simulink model "Lidar_System_FullStateOct25"  (Simulink 7.3)
settings: Solver=FixedStepDiscrete  StartTime=0.0  StopTime=inf  FixedStep=0.1  MaxStep=0.2  RelTol=1e-3
undefined symbols (not defined in the file): strel
libraries: dspmtrx3 x28, simulink x13, dspstat3 x10, vipstatistics x7, vipmorphops x7, dspindex x1
(part 3 of 3)

== matlab function Enabled Subsystem1/Perception/Color Analysis/Docking (Circle)/Docking1/Recognition/Embedded MATLAB Function ==
  data: targetTemp input double; bbox_out output double; cruciform input double; circle input double; triangle input double; whitePixCount input double; threshold input double; V_mask input double; bbox_in input double; returnRatioDiff output double
function [bbox_out,returnRatioDiff] = recognition(targetTemp,cruciform,circle,triangle,...
    whitePixCount,threshold,V_mask,bbox_in)

% Written by Edward Zhu on 5/14/14

% Inputs
% tempID:       Number corresponding to one of the templates (cruciform: 1,
%               circle: 2, triangle: 3)
% cruciform:    19*19 template of cruciform
% circle:       19*19 template of circle
% triangle:     19*19 template of triangle
% whitePixCount:Number of white pixels in each of the templates
% V_mask:       V channel binary mask
% bbox_in:      Bounding boxes as found by blob analysis
% label:        Label matrix as found by blob analysis

% Outputs
% bbox_out:     Bounding box of matched symbol
% symFound:     Status of matching (found: 1, not found: 0)

% Define frame and template size
templates = zeros(19,19,3);
templates(:,:,1) = cruciform;
templates(:,:,2) = circle;
templates(:,:,3) = triangle;
templates = 2*(templates-0.5);

tempRows = size(templates,1);
tempCols = size(templates,2);
numBBox = size(bbox_in,1);

% Initialize scaled image and output bbox matrices
V_scaled = zeros(tempRows,tempCols);
bbox_out = uint32(zeros(numBBox,4));

returnRatioDiff = ones(numBBox,1);

for i = 1:numBBox
       
    if (min(bbox_in(i,:)) > 0 && (bbox_in(i,1)+bbox_in(i,3)) < 640  && (bbox_in(i,2) + bbox_in(i,4) < 480))
        similarity = 0;
        rowScaleStep = floor(bbox_in(i,4) / tempRows);
        colScaleStep = floor(bbox_in(i,3) / tempCols);
        
        captureRow = bbox_in(i,2);
        for row = 1:tempRows
            captureCol = bbox_in(i,1);
            if (captureCol > 640)
                captureCol = uint32(640);
            end
            if (captureRow > 480)
                captureRow = uint32(480);
            end
            for col = 1:tempCols
                V_scaled(row,col) = V_mask(captureRow,captureCol);
                similarity = similarity + templates(row,col,targetTemp) * (V_mask(captureRow,captureCol)*(-1) + 1);
                captureCol = captureCol + colScaleStep;
            end
            captureRow = captureRow + rowScaleStep;
        end
        
        ratioDiff = abs(1 - single(similarity) / single(whitePixCount(targetTemp)));
        
        % Output valid bounding box
        if ratioDiff < threshold
            bbox_out(i,:) = bbox_in(i,:);
            returnRatioDiff(i) = ratioDiff;
        end
    end
end

== matlab function Enabled Subsystem1/Perception/Color Analysis/Docking (Cross)/Docking1/Embedded MATLAB Function ==
  data: xRec input double; bayNumber output double; xDet input double
function bayNumber = bayPosition(xRec,xDet)

symxpos = xRec(1);

diff1 = xDet(1) - symxpos;
diff2 = xDet(2) - symxpos;
diff3 = xDet(3) - symxpos;

if diff1 == 0
    bayNumber = uint8(1);
elseif diff2 == 0
    bayNumber = uint8(2);
elseif diff3 == 0
    bayNumber = uint8(3);
else
    bayNumber = uint8(0);
end

== matlab function Enabled Subsystem1/Perception/Color Analysis/Docking (Cross)/Docking1/Embedded MATLAB Function1 ==
  data: uv_d input double; Distances output double; BBox input double; Angles output double
function [Distances, Angles]  = DsitFind(uv_d,BBox)

% Based on the location of the signs find their distance

% Predefine output distance matrix
Distances = zeros(4,1);
Angles = zeros(4,1);

% Parse BBox information
xpos = BBox(1,1);
ypos = BBox(1,2);
width = BBox(1,3);
height = BBox(1,4);

% Zero count and total of distance measurements
count = 0;
total = 0;

for i = ypos:(ypos+height)
    for j = xpos:(xpos+width)
        % Find total number of points in box where distance value has
        % been gathered and total of all distance in box
        if (uv_d(i,j) > 1)
            count = count+1;
            total = total+uv_d(i,j);
        end
    end
end

% Find average value of nonzero elements inside BBox
Distances(1,1) = round(total/(count*10));
Angles(1,1) = ((xpos + width)/2-3.135858904821101e+02)/554.8582*180/pi;


end

== matlab function Enabled Subsystem1/Perception/Color Analysis/Docking (Cross)/Docking1/Recognition/Embedded MATLAB Function ==
  data: targetTemp input double; bbox_out output double; cruciform input double; circle input double; triangle input double; whitePixCount input double; threshold input double; V_mask input double; bbox_in input double; returnRatioDiff output double
function [bbox_out,returnRatioDiff] = recognition(targetTemp,cruciform,circle,triangle,...
    whitePixCount,threshold,V_mask,bbox_in)

% Written by Edward Zhu on 5/14/14

% Inputs
% tempID:       Number corresponding to one of the templates (cruciform: 1,
%               circle: 2, triangle: 3)
% cruciform:    19*19 template of cruciform
% circle:       19*19 template of circle
% triangle:     19*19 template of triangle
% whitePixCount:Number of white pixels in each of the templates
% V_mask:       V channel binary mask
% bbox_in:      Bounding boxes as found by blob analysis
% label:        Label matrix as found by blob analysis

% Outputs
% bbox_out:     Bounding box of matched symbol
% symFound:     Status of matching (found: 1, not found: 0)

% Define frame and template size
templates = zeros(19,19,3);
templates(:,:,1) = cruciform;
templates(:,:,2) = circle;
templates(:,:,3) = triangle;
templates = 2*(templates-0.5);

tempRows = size(templates,1);
tempCols = size(templates,2);
numBBox = size(bbox_in,1);

% Initialize scaled image and output bbox matrices
V_scaled = zeros(tempRows,tempCols);
bbox_out = uint32(zeros(numBBox,4));

returnRatioDiff = ones(numBBox,1);

for i = 1:numBBox
       
    if (min(bbox_in(i,:)) > 0 && (bbox_in(i,1)+bbox_in(i,3)) < 640  && (bbox_in(i,2) + bbox_in(i,4) < 480))
        similarity = 0;
        rowScaleStep = floor(bbox_in(i,4) / tempRows);
        colScaleStep = floor(bbox_in(i,3) / tempCols);
        
        captureRow = bbox_in(i,2);
        for row = 1:tempRows
            captureCol = bbox_in(i,1);
            if (captureCol > 640)
                captureCol = uint32(640);
            end
            if (captureRow > 480)
                captureRow = uint32(480);
            end
            for col = 1:tempCols
                V_scaled(row,col) = V_mask(captureRow,captureCol);
                similarity = similarity + templates(row,col,targetTemp) * (V_mask(captureRow,captureCol)*(-1) + 1);
                captureCol = captureCol + colScaleStep;
            end
            captureRow = captureRow + rowScaleStep;
        end
        
        ratioDiff = abs(1 - single(similarity) / single(whitePixCount(targetTemp)));
        
        % Output valid bounding box
        if ratioDiff < threshold
            bbox_out(i,:) = bbox_in(i,:);
            returnRatioDiff(i) = ratioDiff;
        end
    end
end

== matlab function Enabled Subsystem1/Perception/Color Analysis/Docking (Triangle)/Docking1/BBox Transform ==
  data: BBin input double; BBout output double
function BBout = Btrans(BBin)
%Change BBbox from 2009 layout to 2014 layout to work with other code

BBinT = BBin';

r1 = BBinT(2,:);
c1 = BBinT(1,:);
h1 = BBinT(4,:);
w1 = BBinT(3,:);

% x1 = BBinT(:,2);
% y1 = BBinT(:,1);
% h1 = BBinT(:,3);
% w1 = BBinT(:,4);

BBout = [r1;c1;h1;w1];
%BBout = [x1 y1 w1 h1];

== matlab function Enabled Subsystem1/Perception/Color Analysis/Docking (Triangle)/Docking1/Blob Analysis/BBox Transform ==
  data: BBin input double; BBout output double
function BBout = Btrans(BBin)
%Change BBbox from 2009 layout to 2014 layout to work with other code

BBinT = BBin';

x1 = BBinT(:,2);
y1 = BBinT(:,1);
h1 = BBinT(:,3);
w1 = BBinT(:,4);

BBout = [x1 y1 w1 h1];

== matlab function Enabled Subsystem1/Perception/Color Analysis/Docking (Triangle)/Docking1/Detection/Detection ==
  data: cruciform input double; bbox_out output double; circle input double; triangle input double; whitePixCount input double; threshold input double; V_mask input double; bbox_in input double; label input double; rtnRatioDiff output double
function [bbox_out,rtnRatioDiff]= detection(cruciform,circle,triangle,...
    whitePixCount,threshold,V_mask,bbox_in,label)

% Written by Edward Zhu on 5/14/14

% Inputs
% tempID:       Number corresponding to one of the templates (cruciform: 1,
%               circle: 2, triangle: 3)
% cruciform:    19*19 template of cruciform
% circle:       19*19 template of circle
% triangle:     19*19 template of triangle
% whitePixCount:Number of white pixels in each of the templates
% V_mask:       V channel binary mask
% bbox_in:      Bounding boxes as found by blob analysis
% label:        Label matrix as found by blob analysis

% Outputs
% bbox_out:     Bounding box of matched symbol
% symFound:     Status of matching (found: 1, not found: 0)

% Define frame and template size
templates = zeros(19,19,3);
templates(:,:,1) = cruciform;
templates(:,:,2) = circle;
templates(:,:,3) = triangle;

imgRows = size(label,1);
imgCols = size(label,2);
tempRows = size(templates,1);
tempCols = size(templates,2);
numBBox = size(bbox_in,1);

% Initialize scaled image and output bbox matrices
V_scaled = zeros(tempRows,tempCols);
bbox_out = uint32(zeros(numBBox,4));
rtnRatioDiff = ones(numBBox,1);

bestRatioDiff = single(1);

for i = 1:numBBox
    shapeDiff = abs(1-bbox_in(i,3)/bbox_in(i,4));
    if bbox_in(i,3) >= tempCols && bbox_in(i,4) >= tempRows && shapeDiff < 0.5
        % Set up arrays for the start and end rows and columns for bbox
        % matching
        
        similarity = zeros(1,3);
        ratioDiff = zeros(1,3);
        
        rowStep = floor(bbox_in(i,4) / tempRows);
        colStep = floor(bbox_in(i,3) / tempCols);
        
        startRowList = zeros(1,3);
        startRowList(2) = bbox_in(i,2);
        startRowList(1) = max(1, startRowList(2) - rowStep);
        startRowList(3) = min(imgRows, startRowList(2) + rowStep);
        
        endRowList = zeros(1,3);
        endRowList(2) = bbox_in(i,2) + bbox_in(i,4);
        endRowList(1) = max(1, endRowList(2) - rowStep);
        endRowList(3) = min(imgRows, endRowList(2) + rowStep);
        
        startColList = zeros(1,3);
        startColList(2) = bbox_in(i,1);
        startColList(1) = max(1, startColList(2) - colStep);
        startColList(3) = min(imgCols, startColList(2) + colStep);
        
        endColList = zeros(1,3);
        endColList(2) = bbox_in(i,1) + bbox_in(i,3);
        endColList(1) = max(1, endColList(2) - colStep);
        endColList(3) = min(imgCols, endColList(2) + colStep);
        
        % Scale down image in bbox to size of template (18*18 px)
        for startRow = startRowList
            for endRow = endRowList
                rowScaleStep = floor((endRow - startRow) / tempRows);
                
                for startCol = startColList
                    for endCol = endColList
                        colScaleStep = floor((endCol - startCol) / tempCols);
                        
                        captureRow = startRow;
                        for row = 1:tempRows
                            captureCol = startCol;
                            for col = 1:tempCols
                                V_scaled(row,col) = V_mask(captureRow,captureCol);
                                for tempID = 1:3
                                    similarity(tempID) = similarity(tempID) + templates(row,col,tempID) * (V_mask(captureRow,captureCol)*(-1) + 1);
                                end
                                captureCol = captureCol + colScaleStep;                        
                            end
                            captureRow = captureRow + rowScaleStep;
                        end                  
                        
                        for tempID = 1:3   
                            ratioDiff(tempID) = abs(1 - single(similarity(tempID)) / single(whitePixCount(tempID))); 
                        end
                        
                        if min(ratioDiff) < bestRatioDiff
                            bestRatioDiff = single(min(ratioDiff));
                        end
                    end
                end
            end
        end
        
        % Output valid bounding boxes
        if bestRatioDiff < threshold
            bbox_out(i,:) = bbox_in(i,:);
            rtnRatioDiff(i) = bestRatioDiff;
        end
    end
end

== matlab function Enabled Subsystem1/Perception/Color Analysis/Docking (Triangle)/Docking1/Embedded MATLAB Function ==
  data: xRec input double; bayNumber output double; xDet input double
function bayNumber = bayPosition(xRec,xDet)

symxpos = xRec(1);

diff1 = xDet(1) - symxpos;
diff2 = xDet(2) - symxpos;
diff3 = xDet(3) - symxpos;

if diff1 == 0
    bayNumber = uint8(1);
elseif diff2 == 0
    bayNumber = uint8(2);
elseif diff3 == 0
    bayNumber = uint8(3);
else
    bayNumber = uint8(0);
end

== matlab function Enabled Subsystem1/Perception/Color Analysis/Docking (Triangle)/Docking1/Embedded MATLAB Function1 ==
  data: uv_d input double; Distances output double; BBox input double; Angles output double
function [Distances, Angles]  = DsitFind(uv_d,BBox)

% Based on the location of the signs find their distance

% Predefine output distance matrix
Distances = zeros(4,1);
Angles = zeros(4,1);

% Parse BBox information
xpos = BBox(1,1);
ypos = BBox(1,2);
width = BBox(1,3);
height = BBox(1,4);

% Zero count and total of distance measurements
count = 0;
total = 0;

for i = ypos:(ypos+height)
    for j = xpos:(xpos+width)
        % Find total number of points in box where distance value has
        % been gathered and total of all distance in box
        if (uv_d(i,j) > 1)
            count = count+1;
            total = total+uv_d(i,j);
        end
    end
end

% Find average value of nonzero elements inside BBox
Distances(1,1) = round(total/(count*10));
Angles(1,1) = ((xpos + width)/2-3.135858904821101e+02)/554.8582*180/pi;


end

== matlab function Enabled Subsystem1/Perception/Color Analysis/Docking (Triangle)/Docking1/Recognition/Embedded MATLAB Function ==
  data: targetTemp input double; bbox_out output double; cruciform input double; circle input double; triangle input double; whitePixCount input double; threshold input double; V_mask input double; bbox_in input double; returnRatioDiff output double
function [bbox_out,returnRatioDiff] = recognition(targetTemp,cruciform,circle,triangle,...
    whitePixCount,threshold,V_mask,bbox_in)

% Written by Edward Zhu on 5/14/14

% Inputs
% tempID:       Number corresponding to one of the templates (cruciform: 1,
%               circle: 2, triangle: 3)
% cruciform:    19*19 template of cruciform
% circle:       19*19 template of circle
% triangle:     19*19 template of triangle
% whitePixCount:Number of white pixels in each of the templates
% V_mask:       V channel binary mask
% bbox_in:      Bounding boxes as found by blob analysis
% label:        Label matrix as found by blob analysis

% Outputs
% bbox_out:     Bounding box of matched symbol
% symFound:     Status of matching (found: 1, not found: 0)

% Define frame and template size
templates = zeros(19,19,3);
templates(:,:,1) = cruciform;
templates(:,:,2) = circle;
templates(:,:,3) = triangle;
templates = 2*(templates-0.5);

tempRows = size(templates,1);
tempCols = size(templates,2);
numBBox = size(bbox_in,1);

% Initialize scaled image and output bbox matrices
V_scaled = zeros(tempRows,tempCols);
bbox_out = uint32(zeros(numBBox,4));

returnRatioDiff = ones(numBBox,1);

for i = 1:numBBox
       
    if (min(bbox_in(i,:)) > 0 && (bbox_in(i,1)+bbox_in(i,3)) < 640  && (bbox_in(i,2) + bbox_in(i,4) < 480))
        similarity = 0;
        rowScaleStep = floor(bbox_in(i,4) / tempRows);
        colScaleStep = floor(bbox_in(i,3) / tempCols);
        
        captureRow = bbox_in(i,2);
        for row = 1:tempRows
            captureCol = bbox_in(i,1);
            if (captureCol > 640)
                captureCol = uint32(640);
            end
            if (captureRow > 480)
                captureRow = uint32(480);
            end
            for col = 1:tempCols
                V_scaled(row,col) = V_mask(captureRow,captureCol);
                similarity = similarity + templates(row,col,targetTemp) * (V_mask(captureRow,captureCol)*(-1) + 1);
                captureCol = captureCol + colScaleStep;
            end
            captureRow = captureRow + rowScaleStep;
        end
        
        ratioDiff = abs(1 - single(similarity) / single(whitePixCount(targetTemp)));
        
        % Output valid bounding box
        if ratioDiff < threshold
            bbox_out(i,:) = bbox_in(i,:);
            returnRatioDiff(i) = ratioDiff;
        end
    end
end

== matlab function Enabled Subsystem1/Perception/Color Analysis/Light Buoy/Color Detection/Embedded MATLAB Function ==
  data: BBox input double; Hin input double; ColorOut output double
function ColorOut = ColorA(BBox,Hin)
% Determine color 

% Used to generate image to check if correct
% RMask = zeros(480,640);
% GMask = zeros(480,640);
% BMask = zeros(480,640);

% Obtain upper left row and column, 
% and height and width of Bounding Box
row = BBox(1);
column = BBox(2);
height = BBox(3);
width = BBox(4);

R_Count = 0;
G_Count = 0;
B_Count = 0;
ColorOut = 0;

startrow = row;
startcol = column;
endrow = row + height;
endcol = column + width;

% Ensure bounding box is not outside frame
rowsize = size(Hin,1);
colsize = size(Hin,2);

% Start of box
if (startrow < 1)
    startrow = int32(1);
end
if (startcol < 1)
    startcol = int32(1);
end
%End of box
if (endrow > rowsize)
    endrow = int32(rowsize);
end
if (endcol > colsize)
    endcol = int32(colsize);
end

% Check for color within Bounding Box
for i = startrow:endrow
    for j = startcol:endcol
        
        % Create Red Image
        if (Hin(i,j) >= 250 || Hin(i,j) < 4)
            %RMask(i,j) = 1;
            R_Count = R_Count+1;
        end
        
        % Create Green Image
        if (Hin(i,j) > 75 && Hin(i,j) < 95)
            %GMask(i,j) = 1;
            G_Count = G_Count+1;
        end
        
        % Create Blue Image
        if (Hin(i,j) > 160 && Hin(i,j) < 175)
            %BMask(i,j) = 1;
            B_Count = B_Count+1;
        end
        
    end
end

if (R_Count > 30)
    ColorOut = 1;
elseif (G_Count > 30)
    ColorOut = 2;
elseif (B_Count > 30)
    ColorOut = 3;
else
    ColorOut = 0;
end

== matlab function Enabled Subsystem1/Perception/Color Analysis/Light Buoy/Format ==
  data: ColorOut input double; Color output double
function Color = CForm(ColorOut)

% Take output of Light Buoy Analysis and put it into the 
% Required from to Communicate with PandaBoard

Color = zeros(4,1);
Color(1,1) = ColorOut(1,1);
Color(2,1) = ColorOut(2,1);
Color(3,1) = ColorOut(3,1);

if (Color(1,1) > 0 && ColorOut(2,1) > 0 && ColorOut(3,1) >0)
    Color(4,1) = 1;
end

== matlab function Enabled Subsystem1/Perception/Detect Landmarks/Subsystem1/Embedded MATLAB Function1 ==
  data: Distances output double; Angles output double
function [Distances, Angles] = landmarkInfo()
%Written by Anderson Lebbad on July 22, 2014
%Last Edited:

%This function finds the average depth of a detected blob and the relative
%angle of it

%Initialize variables
numBlobs = 12;
Distances = zeros(1,numBlobs);
Angles = zeros(1,numBlobs);

end
